simulink model "p5p5e_wave_influence_mod"  (Simulink 9.2)
settings: Solver=ode45  StartTime=0.0  StopTime=1000  RelTol=1e-3  EnableMultiTasking=on
undefined symbols (not defined in the file or in its folder): K_pd, S_t, T_d, T_f
libraries: simulink x2
settings Model: Creator=markh  LastModifiedBy=Martin
settings DataIOCC: SignalLoggingName=sigsOut
settings OptimizationCC: InitFltsAndDblsToZero=on
settings DebuggingCC: SaveWithParameterizedLinksMsg=none  SignalResolutionControl=TryResolveAllWithWarning  MultiTaskDSMMsg=warning  MultiTaskCondExecSysMsg=none  LibraryContextMissingDiagnostic=none
settings HardwareCC: TargetUnknown=on
settings GRTTargetCC: TargetFcnLib=ansi_tfl_tmw.mat

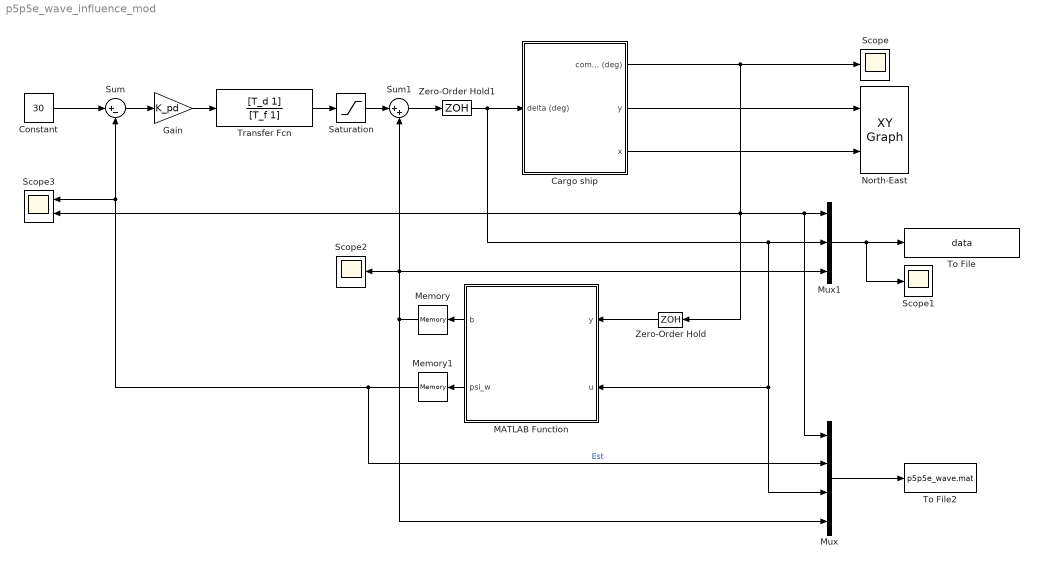
== system p5p5e_wave_influence_mod ==
  Cargo ship : Subsystem  mask(Simple shipmodel for a cargo ship){noise=off, current=off, logic=on}
      mask prompts: noise "measurement noise"; logic "waves"
      mask help:
      | Measurement noise:
      | 	checked = noise on
      | 	unchecked = noise off
      |
      | Current:
      | 	checked = current on
      | 	unchecked = current off
      |
      | Waves:
      | 	checked = waves on
      | 	unchecked = waves off
      |
      | Author: J�rgen Spj�tvold, 9/10-2003
      | TTK 4115 Linear system theory.
      | Modified by Jostein Bakkeheim 26/10-2006
  Constant : Constant  Value=30
  Gain : Gain  Gain=K_pd
  MATLAB Function : MATLAB Function  TreatAsAtomicUnit=on
  Memory : Memory
  Memory1 : Memory
  Mux : Mux
  Mux1 : Mux  Inputs=3
  North-East : simulink/Sinks/XY Graph  xmin=-5000  xmax=5000  ymin=-5000  ymax=5000  st=-1
  Saturation : Saturate  UpperLimit=35  LowerLimit=-35
  Scope : Scope
  Scope1 : Scope
  Scope2 : Scope
  Scope3 : Scope  NumInputPorts=2
  Sum : Sum  Inputs=|+-
  Sum1 : Sum  Inputs=|++
  To File : ToFile  Filename=data  MatrixName=data  SaveFormat=Timeseries
  To File2 : ToFile  Filename=p5p5e_wave.mat
  Transfer Fcn : TransferFcn  Numerator=[T_d 1]  Denominator=[T_f 1]
  Zero-Order Hold : ZeroOrderHold  SampleTime=S_t
  Zero-Order Hold1 : ZeroOrderHold  SampleTime=S_t
  wires:
  Sum1/1 -> Zero-Order Hold1/1
  Cargo ship/1(compass (deg)) -> Scope3/2, Zero-Order Hold/1, Mux/1, Mux1/1, Scope/1
  Zero-Order Hold/1 -> MATLAB Function/1(y)
  MATLAB Function/1(b) -> Memory/1
  Constant/1 -> Sum/1
  Zero-Order Hold1/1 -> Mux1/2, MATLAB Function/2(u), Mux/3, Cargo ship/1(delta (deg))
  Mux1/1 -> To File/1, Scope1/1
  Memory1/1 -> Mux/2, Sum/2, Scope3/1  "Est"
  Cargo ship/3(x) -> North-East/2
  Cargo ship/2(y) -> North-East/1
  MATLAB Function/2(psi_w) -> Memory1/1
  Gain/1 -> Transfer Fcn/1
  Saturation/1 -> Sum1/1
  Memory/1 -> Sum1/2, Scope2/1, Mux1/3, Mux/4
  Sum/1 -> Gain/1
  Transfer Fcn/1 -> Saturation/1
  Mux/1 -> To File2/1

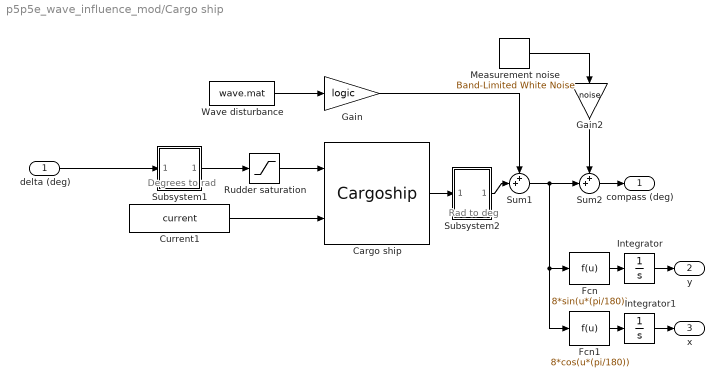
== system p5p5e_wave_influence_mod/Cargo ship ==
  note: Degrees to rad
  note: Rad to deg
  delta (deg) : Inport
  Cargo ship : S-Function  FunctionName=Cargoship  SFunctionDeploymentMode=off  EnableBusSupport=off  mask(Cargo ship){}
      mask help:
      | S-function which simulates a cargo ship.
      |
      | Author: J�rgen Spj�tvold
      | 20.10-2003
      | Modified by Jostein Bakkeheim 27.10.2006
  Current1 : Constant  Value=current
  Fcn : Fcn  Expr=8*sin(u*(pi/180))
  Fcn1 : Fcn  Expr=8*cos(u*(pi/180))
  Gain : Gain  Gain=logic  SaturateOnIntegerOverflow=on  OutDataTypeStr=Inherit: Same as input  ParamDataTypeStr=Inherit: Same as input
  Gain2 : Gain  Gain=noise  SaturateOnIntegerOverflow=on  OutDataTypeStr=Inherit: Same as input  ParamDataTypeStr=Inherit: Same as input
  Integrator : Integrator
  Integrator1 : Integrator
  Measurement noise : simulink/Sources/Band-Limited White Noise  Cov=[0.001]  Ts=.5  seed=[23341]
  Rudder saturation : Saturate  UpperLimit=45*(pi/180)  LowerLimit=-45*(pi/180)
  Subsystem1 : Subsystem  mask(degrees to radians){}
      mask help: Converts degrees to radians
      mask Display: fprintf('D2R');
  Subsystem2 : Subsystem  mask(radians to degrees){}
      mask help: Converts radians to degrees
      mask Display: fprintf('R2D');
  Sum1 : Sum  Inputs=++|  SaturateOnIntegerOverflow=on
  Sum2 : Sum  Inputs=++|  SaturateOnIntegerOverflow=on
  Wave disturbance : FromFile  FileName=wave.mat  SampleTime=0
  compass (deg) : Outport
  y : Outport  Port=2
  x : Outport  Port=3
  wires:
  delta (deg)/1 -> Subsystem1/1(In1)
  Fcn/1 -> Integrator/1
  Integrator/1 -> y/1
  Fcn1/1 -> Integrator1/1
  Integrator1/1 -> x/1
  Wave disturbance/1 -> Gain/1
  Subsystem2/1(Out1) -> Sum1/2
  Gain/1 -> Sum1/1
  Sum1/1 -> Fcn/1, Fcn1/1, Sum2/2
  Cargo ship/1 -> Subsystem2/1(In1)
  Subsystem1/1(Out1) -> Rudder saturation/1
  Rudder saturation/1 -> Cargo ship/1
  Sum2/1 -> compass (deg)/1
  Measurement noise/1 -> Gain2/1
  Gain2/1 -> Sum2/1
  Current1/1 -> Cargo ship/2

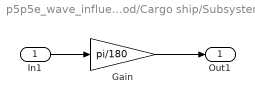
== system p5p5e_wave_influence_mod/Cargo ship/Subsystem1 ==
  In1 : Inport
  Gain : Gain  Gain=pi/180  SaturateOnIntegerOverflow=on  OutDataTypeStr=Inherit: Same as input  ParamDataTypeStr=Inherit: Same as input
  Out1 : Outport
  wires:
  Gain/1 -> Out1/1
  In1/1 -> Gain/1

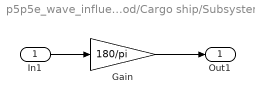
== system p5p5e_wave_influence_mod/Cargo ship/Subsystem2 ==
  In1 : Inport
  Gain : Gain  Gain=180/pi  SaturateOnIntegerOverflow=on  OutDataTypeStr=Inherit: Same as input  ParamDataTypeStr=Inherit: Same as input
  Out1 : Outport
  wires:
  Gain/1 -> Out1/1
  In1/1 -> Gain/1

== matlab function MATLAB Function ==
  data: y input double; b output double; psi_w output double; u input double; data parameter double
function [b, psi_w] = kalman(y,u,data)

persistent init A_d B_d C_d E_d Q R P_min_0 x_min_0 I

if isempty(init)
    init = 1;
    [A_d, B_d, C_d, E_d, Q, R, P_min_0, x_min_0, I] = deal(data.A_d,data.B_d,data.C_d,data.E_d,data.Q,data.R,data.P_min_0,data.x_min_0,data.I);
end

K_k = P_min_0*C_d'*inv((C_d*P_min_0*C_d'+R));

x_k = x_min_0+K_k*(y-C_d*x_min_0);

P_k = (I-K_k*C_d)*P_min_0*((I-K_k*C_d)')+K_k*R*K_k';

x_min_0 = A_d*x_k+B_d*u;

P_min_0  = A_d*P_k*(A_d)'+E_d*Q*(E_d)';

b = x_k(5);
psi_w = x_k(2);

end
